simulink model "fullSystemwSmarttank"  (R2020a)
settings: Solver=VariableStepAuto  StartTime=0.0  StopTime=359  RelTol=1e-3
values from neighbouring files (symbols this model uses):
  basin1 = 55560000    [data.mat]
  k = 1    [data.mat]
  n = 0.02    [data.mat]
  R = 0.75    [data.mat]
  S = 0.2    [data.mat]
libraries: simulink x8
settings Model: Creator=valstandard  LastModifiedBy=lydialagorga
settings SolverCC: AlgebraicLoopSolver=LineSearch

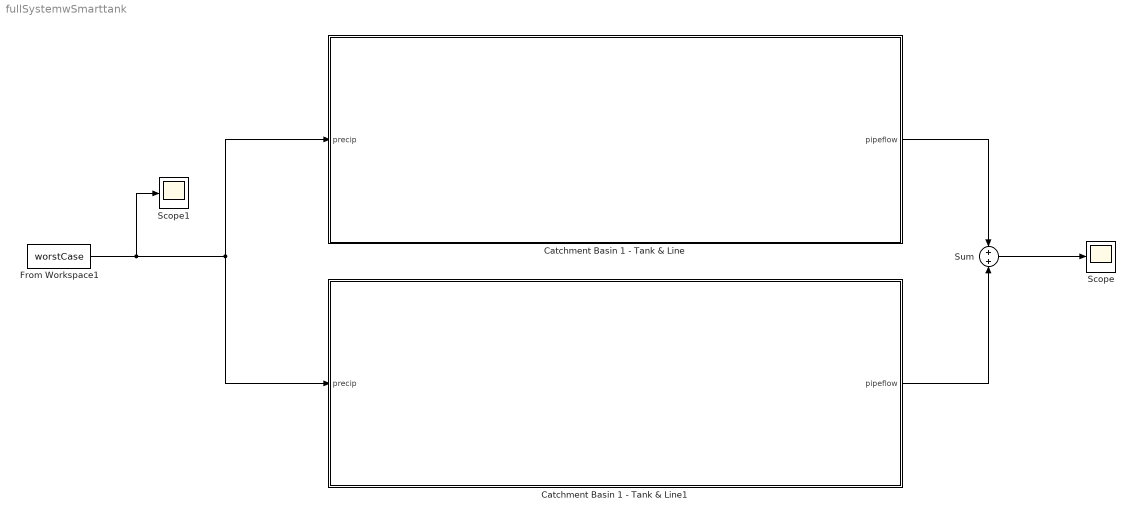
== system fullSystemwSmarttank ==
  Catchment Basin 1 - Tank & Line : Subsystem
  Catchment Basin 1 - Tank & Line1 : Subsystem
  From Workspace1 : FromWorkspace  VariableName=worstCase  SampleTime=1
  Scope : Scope
  Scope1 : Scope
  Sum : Sum  Inputs=+|+
  wires:
  Catchment Basin 1 - Tank & Line1/1(pipeflow) -> Sum/2
  Catchment Basin 1 - Tank & Line/1(pipeflow) -> Sum/1
  Sum/1 -> Scope/1
  From Workspace1/1 -> Catchment Basin 1 - Tank & Line1/1(precip), Catchment Basin 1 - Tank & Line/1(precip), Scope1/1

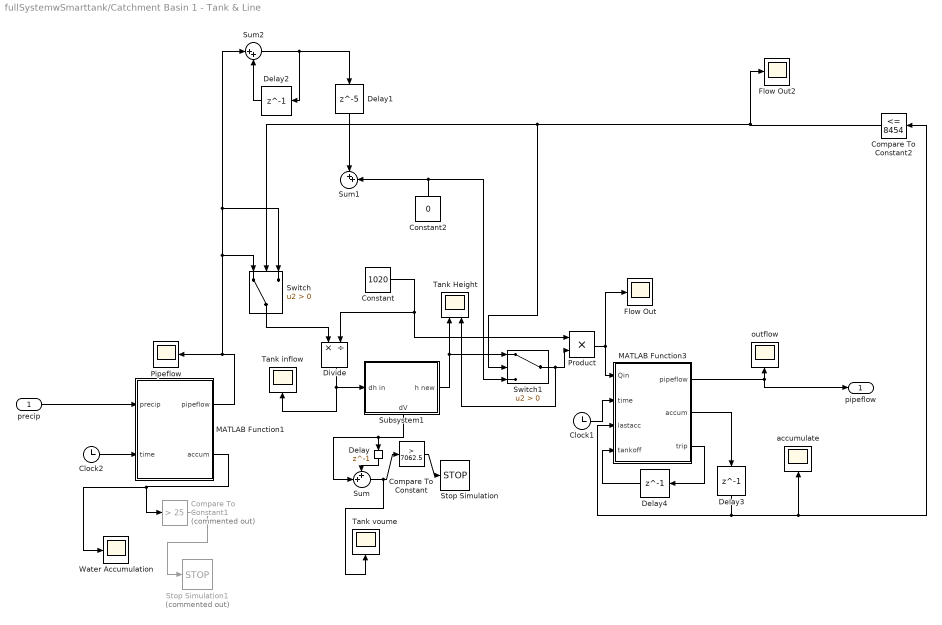
== system fullSystemwSmarttank/Catchment Basin 1 - Tank & Line ==
  precip : Inport
  " Pipeflow" : Scope
  Clock1 : Clock
  Clock2 : Clock
  Compare To Constant : simulink/Logic and Bit Operations/Compare To Constant  relop=>  const=7062.5  OutDataTypeStr=boolean
  Compare To Constant1 : simulink/Logic and Bit Operations/Compare To Constant  Commented=on  relop=>  const=25  OutDataTypeStr=boolean
  Compare To Constant2 : simulink/Logic and Bit Operations/Compare To Constant  relop=<=  const=8454  OutDataTypeStr=boolean
  Constant : Constant  Value=1020
  Constant2 : Constant  Value=0  SampleTime=1
  Delay{,2..4} (4 alike) : Delay  DelayLength=1  InitialCondition=0
  Delay1 : Delay  DelayLength=5  InitialCondition=0
  Divide : Product  Inputs=*/
  Flow Out : Scope
  Flow Out2 : Scope
  MATLAB Function1 : MATLAB Function  TreatAsAtomicUnit=on
  MATLAB Function3 : MATLAB Function  TreatAsAtomicUnit=on
  Product : Product
  Stop Simulation : Stop
  Stop Simulation1 : Stop  Commented=on
  Subsystem1 : Subsystem
      settings: PortSchema="{\"entries\":[{\"content\":{\"sides\":[{\"content\":{\"connectorIds\":[\"In1\"]},\"type\":\"ConnectorPlacement.EquallySpacedRectSide\",\"uuid\":\"49521410-f26e-428f-a0f4-6065ef8c5de4\"},{\"content\":{\"connectorIds\":[\"Out1\"],\"side\":\"RIGHT\"},\"type\":\"ConnectorPlacement.EquallySpacedRectSide\",\"uuid\":\"23e51712-c361-47eb-a12a-34fba58dacf0\"},{\"content\":{\"connectorIds\":[],\"side\":\"TOP\"},\"type\":\"ConnectorPlacement.EquallySpacedRectSide\",\"uuid\":\"3d891762-d113-46ae-9add-fc9d38759335\"},{\"content\":{\"connectorIds\":[\"Out2\"],\"side\":\"BOTTOM\"},\"type\":\"ConnectorPlacement.EquallySpacedRectSide\",\"uuid\":\"478163d5-2f8e-48b3-a9ce-7bd7e130e649\"}]},\"type\":\"ConnectorPlacement.EquallySpacedConnector\",\"uuid\":\"d8b883b0-28bd-4a78-a85b-3cb93156455b\"}],\"packageUris\":[\"http://schema.mathworks.com/mf0/Connector/19700101\"],\"version\":\"1.0\"}"
  Sum : Sum  Inputs=++|
  Sum1 : Sum  Inputs=++|
  Sum2 : Sum  Inputs=|++
  Switch : Switch  Criteria=u2 > Threshold
  Switch1 : Switch  Criteria=u2 > Threshold
  Tank Height : Scope  NumInputPorts=2
  Tank inflow : Scope
  Tank voume : Scope
  Water Accumulation : Scope
  accumulate : Scope
  outflow : Scope
  pipeflow : Outport
  wires:
  Sum/1 -> Tank voume/1, Compare To Constant/1
  MATLAB Function3/1(pipeflow) -> pipeflow/1, outflow/1
  Compare To Constant/1 -> Stop Simulation/1
  Clock2/1 -> MATLAB Function1/2(time)
  precip/1 -> MATLAB Function1/1(precip)
  MATLAB Function3/2(accum) -> Delay3/1
  Product/1 -> Flow Out/1, MATLAB Function3/1(Qin)
  MATLAB Function1/2(accum) -> Water Accumulation/1, Compare To Constant1/1
  Constant/1 -> Product/1, Divide/2
  Subsystem1/1(h new) -> Switch1/1, Tank Height/1
  Delay/1 -> Sum/1
  Subsystem1/2(dV) -> Sum/2, Delay/1
  Clock1/1 -> MATLAB Function3/2(time)
  Compare To Constant1/1 -> Stop Simulation1/1
  Switch1/1 -> Product/2, Tank Height/2
  Compare To Constant2/1 -> Flow Out2/1, Switch/2, Switch1/2
  Divide/1 -> Tank inflow/1, Subsystem1/1(dh in)
  Switch/1 -> Divide/1
  Delay1/1 -> Sum1/1
  Delay2/1 -> Sum2/2
  Sum2/1 -> Delay2/1, Delay1/1
  Constant2/1 -> Sum1/2, Switch1/3
  Delay3/1 -> accumulate/1, Compare To Constant2/1, MATLAB Function3/3(lastacc)
  MATLAB Function1/1(pipeflow) -> " Pipeflow"/1, Switch/3, Sum2/1, Switch/1
  MATLAB Function3/3(trip) -> Delay4/1
  Delay4/1 -> MATLAB Function3/4(tankoff)

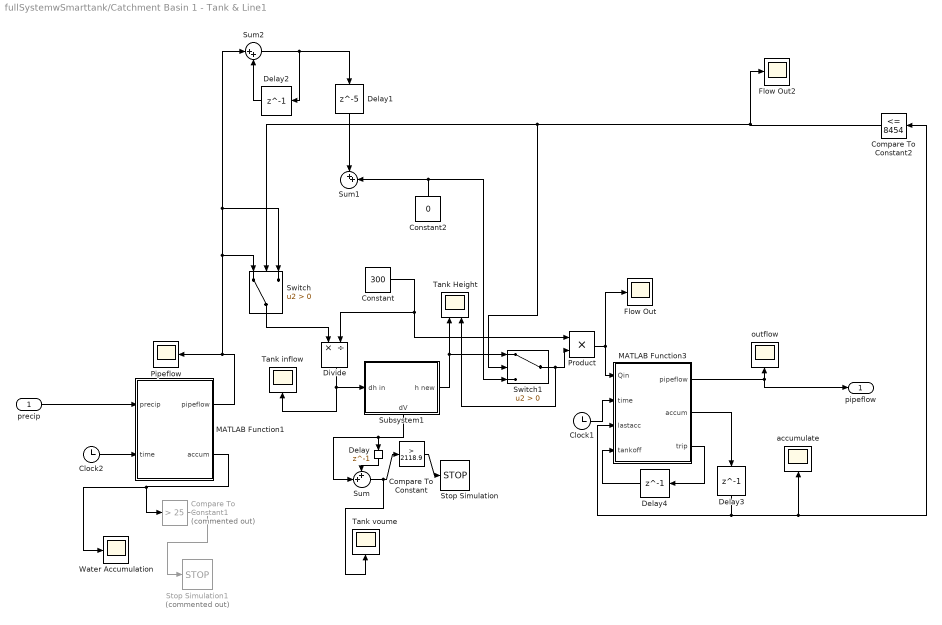
== system fullSystemwSmarttank/Catchment Basin 1 - Tank & Line1 ==
  precip : Inport
  " Pipeflow" : Scope
  Clock1 : Clock
  Clock2 : Clock
  Compare To Constant : simulink/Logic and Bit Operations/Compare To Constant  relop=>  const=2118.9  OutDataTypeStr=boolean
  Compare To Constant1 : simulink/Logic and Bit Operations/Compare To Constant  Commented=on  relop=>  const=25  OutDataTypeStr=boolean
  Compare To Constant2 : simulink/Logic and Bit Operations/Compare To Constant  relop=<=  const=8454  OutDataTypeStr=boolean
  Constant : Constant  Value=300
  Constant2 : Constant  Value=0  SampleTime=1
  Delay{,2..4} (4 alike) : Delay  DelayLength=1  InitialCondition=0
  Delay1 : Delay  DelayLength=5  InitialCondition=0
  Divide : Product  Inputs=*/
  Flow Out : Scope
  Flow Out2 : Scope
  MATLAB Function1 : MATLAB Function  TreatAsAtomicUnit=on
  MATLAB Function3 : MATLAB Function  TreatAsAtomicUnit=on
  Product : Product
  Stop Simulation : Stop
  Stop Simulation1 : Stop  Commented=on
  Subsystem1 : Subsystem
      settings: PortSchema="{\"entries\":[{\"content\":{\"sides\":[{\"content\":{\"connectorIds\":[\"In1\"]},\"type\":\"ConnectorPlacement.EquallySpacedRectSide\",\"uuid\":\"49521410-f26e-428f-a0f4-6065ef8c5de4\"},{\"content\":{\"connectorIds\":[\"Out1\"],\"side\":\"RIGHT\"},\"type\":\"ConnectorPlacement.EquallySpacedRectSide\",\"uuid\":\"23e51712-c361-47eb-a12a-34fba58dacf0\"},{\"content\":{\"connectorIds\":[],\"side\":\"TOP\"},\"type\":\"ConnectorPlacement.EquallySpacedRectSide\",\"uuid\":\"3d891762-d113-46ae-9add-fc9d38759335\"},{\"content\":{\"connectorIds\":[\"Out2\"],\"side\":\"BOTTOM\"},\"type\":\"ConnectorPlacement.EquallySpacedRectSide\",\"uuid\":\"478163d5-2f8e-48b3-a9ce-7bd7e130e649\"}]},\"type\":\"ConnectorPlacement.EquallySpacedConnector\",\"uuid\":\"d8b883b0-28bd-4a78-a85b-3cb93156455b\"}],\"packageUris\":[\"http://schema.mathworks.com/mf0/Connector/19700101\"],\"version\":\"1.0\"}"
  Sum : Sum  Inputs=++|
  Sum1 : Sum  Inputs=++|
  Sum2 : Sum  Inputs=|++
  Switch : Switch  Criteria=u2 > Threshold
  Switch1 : Switch  Criteria=u2 > Threshold
  Tank Height : Scope  NumInputPorts=2
  Tank inflow : Scope
  Tank voume : Scope
  Water Accumulation : Scope
  accumulate : Scope
  outflow : Scope
  pipeflow : Outport
  wires:
  Sum/1 -> Tank voume/1, Compare To Constant/1
  MATLAB Function3/1(pipeflow) -> pipeflow/1, outflow/1
  Compare To Constant/1 -> Stop Simulation/1
  Clock2/1 -> MATLAB Function1/2(time)
  precip/1 -> MATLAB Function1/1(precip)
  MATLAB Function3/2(accum) -> Delay3/1
  Product/1 -> Flow Out/1, MATLAB Function3/1(Qin)
  MATLAB Function1/2(accum) -> Water Accumulation/1, Compare To Constant1/1
  Constant/1 -> Product/1, Divide/2
  Subsystem1/1(h new) -> Switch1/1, Tank Height/1
  Delay/1 -> Sum/1
  Subsystem1/2(dV) -> Sum/2, Delay/1
  Clock1/1 -> MATLAB Function3/2(time)
  Compare To Constant1/1 -> Stop Simulation1/1
  Switch1/1 -> Product/2, Tank Height/2
  Compare To Constant2/1 -> Flow Out2/1, Switch/2, Switch1/2
  Divide/1 -> Tank inflow/1, Subsystem1/1(dh in)
  Switch/1 -> Divide/1
  Delay1/1 -> Sum1/1
  Delay2/1 -> Sum2/2
  Sum2/1 -> Delay2/1, Delay1/1
  Constant2/1 -> Sum1/2, Switch1/3
  Delay3/1 -> accumulate/1, Compare To Constant2/1, MATLAB Function3/3(lastacc)
  MATLAB Function1/1(pipeflow) -> " Pipeflow"/1, Switch/3, Sum2/1, Switch/1
  MATLAB Function3/3(trip) -> Delay4/1
  Delay4/1 -> MATLAB Function3/4(tankoff)

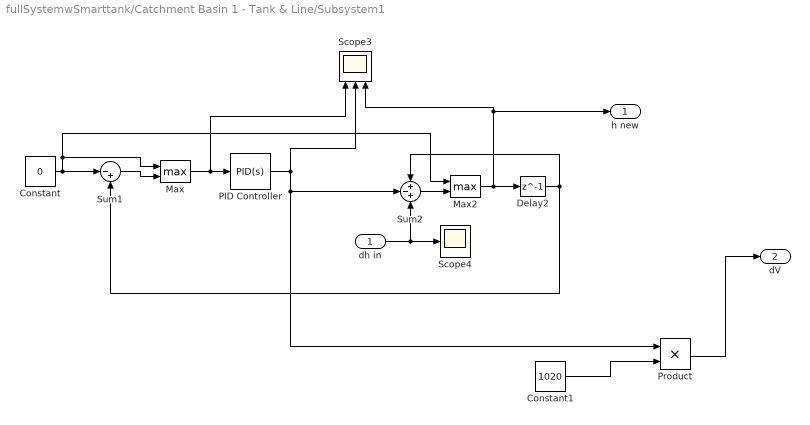
== system fullSystemwSmarttank/Catchment Basin 1 - Tank & Line/Subsystem1 ==
  dh in : Inport
  Constant : Constant  Value=0
  Constant1 : Constant  Value=1020
  Delay2 : Delay  DelayLength=1  InitialCondition=0
  Max : MinMax  Function=max  Inputs=2
  Max2 : MinMax  Function=max  Inputs=2
  PID Controller : simulink/Continuous/PID Controller  Controller=PID  Form=Ideal  TimeDomain=Continuous-time  UseExternalTs=off  SampleTime=-1  IntegratorMethod=Forward Euler  FilterMethod=Forward Euler  ControllerParametersSource=internal  P=0.2  I=0.001  D=.001  UseFilter=on  N=50  TunerSelectOption=Transfer Function Based (PID Tuner App)  InitialConditionSource=internal  InitialConditionForIntegrator=0  InitialConditionForFilter=0  DifferentiatorICPrevScaledInput=0  ExternalReset=none  TrackingMode=off  Kt=1  LimitOutput=on  UpperSaturationLimit=inf  LowerSaturationLimit=0  LinearizeAsGain=on  AntiWindupMode=none  Kb=1  POutMin=0  POutMax=[]  IOutMin=[]  IOutMax=[]  DOutMin=[]  DOutMax=[]  NOutMin=[]  NOutMax=[]  SumOutMin=[]  SumOutMax=[]  SaturationOutMin=[]  SaturationOutMax=[]  PParamMin=[]  PParamMax=[]  IParamMin=[]  IParamMax=[]  DParamMin=[]  DParamMax=[]  NParamMin=[]  NParamMax=[]  KbParamMin=[]  KbParamMax=[]  KtParamMin=[]  KtParamMax=[]  KbOutMin=[]  KbOutMax=[]  KtOutMin=[]  KtOutMax=[]  IntegratorOutMin=[]  IntegratorOutMax=[]  FilterOutMin=[]  FilterOutMax=[]  SumI1OutMin=[]  SumI1OutMax=[]  SumI2OutMin=[]  SumI2OutMax=[]  SumI3OutMin=[]  SumI3OutMax=[]  SumI4OutMin=[]  SumI4OutMax=[]  SumDOutMin=[]  SumDOutMax=[]  DifferentiatorOutMin=[]  DifferentiatorOutMax=[]  FilterDiffOutCoefMin=[]  FilterDiffOutCoefMax=[]  ReciprocalOutMin=[]  ReciprocalOutMax=[]  SumDenOutMin=[]  SumDenOutMax=[]  SumNumOutMin=[]  SumNumOutMax=[]  DivideOutMin=[]  DivideOutMax=[]  UdiffTsProdOutMin=[]  UdiffTsProdOutMax=[]  NTsProdOutMin=[]  NTsProdOutMax=[]  UintegralTsProdOutMin=[]  UintegralTsProdOutMax=[]  UngainTsProdOutMin=[]  UngainTsProdOutMax=[]  IntegratorContinuousStateAttributes=''  IntegratorStateMustResolveToSignalObject=off  IntegratorRTWStateStorageClass=Auto  FilterContinuousStateAttributes=''  FilterStateMustResolveToSignalObject=off  FilterRTWStateStorageClass=Auto  ParallelPVariant=Passthrough  IdealPVariant=InternalParameters  IVariant=InternalParameters  DVariant=InternalParameters  IntegratorVariant=Continuous  SatVariant=Enabled  AWVariant=Passthrough  PCopyVariant=Disabled  TRVariant=Disabled  FdbkBlocksVariant=Forward  IdealPFdbkVariant=Disabled  SatFdbkVariant=Disabled  DerivativeFilterVariant=ContFilter  NVariant=InternalParameters  NCopyVariant=Disabled  FilterICVariant=InternalICsFilter  IntegratorICVariant=InternalICs  ExternalResetVariant=Disabled  TRSumVariant=Passthrough  SumFdbkVariant=Disabled  SumVariant=Sum_PID  TsampFilterVariant=InternalTs  TsampNgainVariant=Passthrough  TsampIntegralVariant=Passthrough
  Product : Product
  Scope3 : Scope  NumInputPorts=3
  Scope4 : Scope
  Sum1 : Sum  Inputs=|-+  OutMin=0
  Sum2 : Sum  Inputs=+-+  OutMin=0
  h new : Outport
  dV : Outport  Port=2
  wires:
  Delay2/1 -> Sum1/2, Sum2/1
  Sum1/1 -> Max/2
  Sum2/1 -> Max2/2
  Max/1 -> Scope3/1, PID Controller/1
  Max2/1 -> Scope3/3, h new/1, Delay2/1
  PID Controller/1 -> Product/1, Sum2/2, Scope3/2
  dh in/1 -> Sum2/3, Scope4/1
  Constant/1 -> Sum1/1, Max/1, Max2/1
  Product/1 -> dV/1
  Constant1/1 -> Product/2

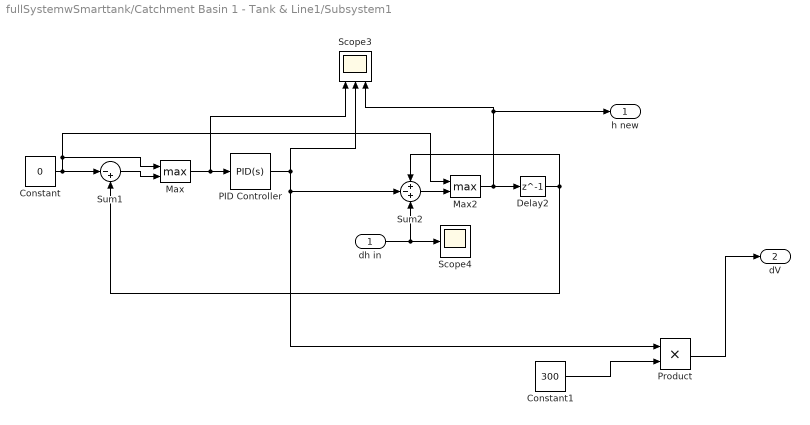
== system fullSystemwSmarttank/Catchment Basin 1 - Tank & Line1/Subsystem1 ==
  dh in : Inport
  Constant : Constant  Value=0
  Constant1 : Constant  Value=300
  Delay2 : Delay  DelayLength=1  InitialCondition=0
  Max : MinMax  Function=max  Inputs=2
  Max2 : MinMax  Function=max  Inputs=2
  PID Controller : simulink/Continuous/PID Controller  Controller=PID  Form=Ideal  TimeDomain=Continuous-time  UseExternalTs=off  SampleTime=-1  IntegratorMethod=Forward Euler  FilterMethod=Forward Euler  ControllerParametersSource=internal  P=0.2  I=0.001  D=.001  UseFilter=on  N=50  TunerSelectOption=Transfer Function Based (PID Tuner App)  InitialConditionSource=internal  InitialConditionForIntegrator=0  InitialConditionForFilter=0  DifferentiatorICPrevScaledInput=0  ExternalReset=none  TrackingMode=off  Kt=1  LimitOutput=on  UpperSaturationLimit=inf  LowerSaturationLimit=0  LinearizeAsGain=on  AntiWindupMode=none  Kb=1  POutMin=0  POutMax=[]  IOutMin=[]  IOutMax=[]  DOutMin=[]  DOutMax=[]  NOutMin=[]  NOutMax=[]  SumOutMin=[]  SumOutMax=[]  SaturationOutMin=[]  SaturationOutMax=[]  PParamMin=[]  PParamMax=[]  IParamMin=[]  IParamMax=[]  DParamMin=[]  DParamMax=[]  NParamMin=[]  NParamMax=[]  KbParamMin=[]  KbParamMax=[]  KtParamMin=[]  KtParamMax=[]  KbOutMin=[]  KbOutMax=[]  KtOutMin=[]  KtOutMax=[]  IntegratorOutMin=[]  IntegratorOutMax=[]  FilterOutMin=[]  FilterOutMax=[]  SumI1OutMin=[]  SumI1OutMax=[]  SumI2OutMin=[]  SumI2OutMax=[]  SumI3OutMin=[]  SumI3OutMax=[]  SumI4OutMin=[]  SumI4OutMax=[]  SumDOutMin=[]  SumDOutMax=[]  DifferentiatorOutMin=[]  DifferentiatorOutMax=[]  FilterDiffOutCoefMin=[]  FilterDiffOutCoefMax=[]  ReciprocalOutMin=[]  ReciprocalOutMax=[]  SumDenOutMin=[]  SumDenOutMax=[]  SumNumOutMin=[]  SumNumOutMax=[]  DivideOutMin=[]  DivideOutMax=[]  UdiffTsProdOutMin=[]  UdiffTsProdOutMax=[]  NTsProdOutMin=[]  NTsProdOutMax=[]  UintegralTsProdOutMin=[]  UintegralTsProdOutMax=[]  UngainTsProdOutMin=[]  UngainTsProdOutMax=[]  IntegratorContinuousStateAttributes=''  IntegratorStateMustResolveToSignalObject=off  IntegratorRTWStateStorageClass=Auto  FilterContinuousStateAttributes=''  FilterStateMustResolveToSignalObject=off  FilterRTWStateStorageClass=Auto  ParallelPVariant=Passthrough  IdealPVariant=InternalParameters  IVariant=InternalParameters  DVariant=InternalParameters  IntegratorVariant=Continuous  SatVariant=Enabled  AWVariant=Passthrough  PCopyVariant=Disabled  TRVariant=Disabled  FdbkBlocksVariant=Forward  IdealPFdbkVariant=Disabled  SatFdbkVariant=Disabled  DerivativeFilterVariant=ContFilter  NVariant=InternalParameters  NCopyVariant=Disabled  FilterICVariant=InternalICsFilter  IntegratorICVariant=InternalICs  ExternalResetVariant=Disabled  TRSumVariant=Passthrough  SumFdbkVariant=Disabled  SumVariant=Sum_PID  TsampFilterVariant=InternalTs  TsampNgainVariant=Passthrough  TsampIntegralVariant=Passthrough
  Product : Product
  Scope3 : Scope  NumInputPorts=3
  Scope4 : Scope
  Sum1 : Sum  Inputs=|-+  OutMin=0
  Sum2 : Sum  Inputs=+-+  OutMin=0
  h new : Outport
  dV : Outport  Port=2
  wires:
  Delay2/1 -> Sum1/2, Sum2/1
  Sum1/1 -> Max/2
  Sum2/1 -> Max2/2
  Max/1 -> Scope3/1, PID Controller/1
  Max2/1 -> Scope3/3, h new/1, Delay2/1
  PID Controller/1 -> Product/1, Sum2/2, Scope3/2
  dh in/1 -> Sum2/3, Scope4/1
  Constant/1 -> Sum1/1, Max/1, Max2/1
  Product/1 -> dV/1
  Constant1/1 -> Product/2

== matlab function fullSystemwSmarttank/Catchment Basin 1 - Tank & Line/MATLAB Function1 ==
  data: pipeflow output; precip input; k parameter; n parameter; R parameter; S parameter; basin1 parameter; time input; accum output
function [pipeflow, accum]  = pipeflow(precip, k, n, R, S, basin1, time)
% v = k*n*R^0.63*S^.54
% cross sectional area: pi*r^2
% v = velocity; n = roughness; R = hydraulic radius; S = slope; k =
% conversions

v = k*n*R^0.63*S^.54; %should be 
Ax = pi*R^2;
pipeflowMax = v*Ax; %pipe flow out is 4.82 m3/s
% if water coming in is below max, it flows in normally
% if above max, then it flows according to the max flow
if precip*basin1 < pipeflowMax
    pipeflow = precip*basin1;
else
    pipeflow = pipeflowMax;
end
accum = precip*basin1*time - pipeflow*time;
end

% h = precip*clock; %calculates the accumulated precipitation
% Qout = C*sqrt(h); 
% dPdt = pipeflow - Qout; %change in volume; 
% % where if dVdt > volume of tank, there's a back up in system
% 
% % dPdt = basin1*precip + wateracc - pipeflow; %water remaining to be assimilated

== matlab function fullSystemwSmarttank/Catchment Basin 1 - Tank & Line1/MATLAB Function1 ==
  data: pipeflow output; precip input; k parameter; n parameter; R parameter; S parameter; basin1 parameter; time input; accum output
function [pipeflow, accum]  = pipeflow(precip, k, n, R, S, basin1, time)
% v = k*n*R^0.63*S^.54
% cross sectional area: pi*r^2
% v = velocity; n = roughness; R = hydraulic radius; S = slope; k =
% conversions

v = k*n*R^0.63*S^.54; %should be 
Ax = pi*R^2;
pipeflowMax = v*Ax; %pipe flow out is 4.82 m3/s
% if water coming in is below max, it flows in normally
% if above max, then it flows according to the max flow
if precip*basin1 < pipeflowMax
    pipeflow = precip*basin1;
else
    pipeflow = pipeflowMax;
end
accum = precip*basin1*time - pipeflow*time;
end

% h = precip*clock; %calculates the accumulated precipitation
% Qout = C*sqrt(h); 
% dPdt = pipeflow - Qout; %change in volume; 
% % where if dVdt > volume of tank, there's a back up in system
% 
% % dPdt = basin1*precip + wateracc - pipeflow; %water remaining to be assimilated

== matlab function fullSystemwSmarttank/Catchment Basin 1 - Tank & Line1/MATLAB Function3 ==
  data: pipeflow output; Qin input; k parameter; n parameter; R parameter; S parameter; time input; accum output; lastacc input; trip output; tankoff input
function [pipeflow, accum,trip] = pipeflow( Qin, k, n, R, S, time,lastacc,tankoff)
v = k*n*R^0.63*S^.54; %ft/s
qmax = v*(pi*R^2);
trip = tankoff;
if Qin < qmax
    pipeflow = Qin;
else
    pipeflow = qmax;
end
accum = max((lastacc + (Qin-qmax)),0);
% if Qin == 0 && lastacc > 0
%     pipeflow = qmax;
%     trip = 1;
% end
% if tankoff == 1
%     lastacc = lastacc-60;
%     accum = lastacc - qmax;
% end

end

== matlab function fullSystemwSmarttank/Catchment Basin 1 - Tank & Line/MATLAB Function3 ==
  data: pipeflow output; Qin input; k parameter; n parameter; R parameter; S parameter; time input; accum output; lastacc input; trip output; tankoff input
function [pipeflow, accum,trip] = pipeflow( Qin, k, n, R, S, time,lastacc,tankoff)
v = k*n*R^0.63*S^.54; %ft/s
qmax = v*(pi*R^2);
trip = tankoff;
if Qin < qmax
    pipeflow = Qin;
else
    pipeflow = qmax;
end
accum = max((lastacc + (Qin-qmax)),0);
% if Qin == 0 && lastacc > 0
%     pipeflow = qmax;
%     trip = 1;
% end
% if tankoff == 1
%     lastacc = lastacc-60;
%     accum = lastacc - qmax;
% end

end
